simulink library "ammclib_bam_S32K3xx"  (R2016a)
settings: Solver=VariableStepAuto  SolverMode=SingleTasking  StartTime=0.0  StopTime=10.0  RelTol=1e-3
undefined symbols (not defined in the file or in its folder): a1, a2, ADCMaxError, autoCalcEn, b0, b1, b2, cfg, dgain, escale, f16A1, f16A2, f16ADCMaxError, f16B0, f16B1, f16B2, f16C1, f16CC1sc, f16CC1sc_D, f16CC1sc_Q, f16CC2sc, f16CC2sc_D, f16CC2sc_Q, f16DerivGain, f16EGain, f16FiltCoef, f16HystOff, f16HystOn, f16IGain, f16IntegGain, f16IntegGain_D, f16IntegGain_Q, f16IntegGainQ, f16Kd, f16KLs, f16Kq, f16KRs, f16Limit, f16LowerLimit, f16LowerLimit_D, f16LowerLimit_Q, f16LowerLimitQ, f16ModIndex, f16OutValOff, f16OutValOn, f16PropGain, f16PropGain_D, f16PropGain_Q, f16PropGainQ, f16RampDown, f16RampUp, f16UGain, f16UpperLimit, f16UpperLimit_D, f16UpperLimit_Q, f16UpperLimitQ, f16WIGain, f32A1, f32A2, f32ADCMaxError ... (+180)
(part 48 of 50)

== system ammclib_bam_S32K3xx/GMCLIB/F32/GMCLIB_SvmU0n_F32 ==
  pIn : Inport  OutDataTypeStr=Bus: SWLIBS_2Syst_F32  BusOutputAsStruct=on
  GMCLIB_SvmU0n_SF : S-Function  FunctionName=GMCLIB_SvmU0n_SF_F32  SFunctionDeploymentMode=off  EnableBusSupport=off
  copyright : Subsystem
      mask Display: text(10,90,'FILE:');text(10,75,'DESRIPTION:');text(10,60,'COPYRIGHT:');text(10,45,'VERSION:');text(10,30,'DATE:')
  copyright2 : Subsystem
      mask Display: text(10,90,'GMCLIB_SvmU0n_BAM_F32.slx');text(10,75,'Special Space Vector Modulation with O_000 Nulls.');text(10,60,'NXP 2022');text(10,45,'1.0');text(10,30,'20-Apr-2022');
  u32Sector : Outport
  pOut : Outport  Port=2
  wires:
  GMCLIB_SvmU0n_SF/2 -> pOut/1
  GMCLIB_SvmU0n_SF/1 -> u32Sector/1
  pIn/1 -> GMCLIB_SvmU0n_SF/1

== system ammclib_bam_S32K3xx/GMCLIB/F32/GMCLIB_SvmU7n_F32 ==
  pIn : Inport  OutDataTypeStr=Bus: SWLIBS_2Syst_F32  BusOutputAsStruct=on
  GMCLIB_SvmU7n_SF : S-Function  FunctionName=GMCLIB_SvmU7n_SF_F32  SFunctionDeploymentMode=off  EnableBusSupport=off
  copyright : Subsystem
      mask Display: text(10,90,'FILE:');text(10,75,'DESRIPTION:');text(10,60,'COPYRIGHT:');text(10,45,'VERSION:');text(10,30,'DATE:')
  copyright2 : Subsystem
      mask Display: text(10,90,'GMCLIB_SvmU7n_BAM_F32.slx');text(10,75,'Special Space Vector Modulation with O_111 Ones.');text(10,60,'NXP 2022');text(10,45,'1.0');text(10,30,'20-Apr-2022');
  u32Sector : Outport
  pOut : Outport  Port=2
  wires:
  GMCLIB_SvmU7n_SF/2 -> pOut/1
  GMCLIB_SvmU7n_SF/1 -> u32Sector/1
  pIn/1 -> GMCLIB_SvmU7n_SF/1

== system ammclib_bam_S32K3xx/GMCLIB/F32/GMCLIB_VRot_F32 ==
  f32InVec : Inport  OutDataTypeStr=Bus: SWLIBS_2Syst_F32  BusOutputAsStruct=on
  f32Angle : Inport  Port=2  OutDataTypeStr=int32
  GMCLIB_VRot_SF : S-Function  FunctionName=GMCLIB_VRot_SF_F32  SFunctionDeploymentMode=off  EnableBusSupport=off
  copyright : Subsystem
      mask Display: text(10,90,'FILE:');text(10,75,'DESRIPTION:');text(10,60,'COPYRIGHT:');text(10,45,'VERSION:');text(10,30,'DATE:')
  copyright2 : Subsystem
      mask Display: text(10,90,'GMCLIB_VRot_BAM_F32.slx');text(10,75,'Vector rotation.');text(10,60,'NXP 2022');text(10,45,'1.0');text(10,30,'20-Apr-2022');
  f32OutVec : Outport
  wires:
  GMCLIB_VRot_SF/1 -> f32OutVec/1
  f32Angle/1 -> GMCLIB_VRot_SF/2
  f32InVec/1 -> GMCLIB_VRot_SF/1

== system ammclib_bam_S32K3xx/GMCLIB/F32/GMCLIB_VUnit_F32 ==
  f32InVec : Inport  OutDataTypeStr=Bus: SWLIBS_2Syst_F32  BusOutputAsStruct=on
  GMCLIB_VUnit_SF : S-Function  FunctionName=GMCLIB_VUnit_SF_F32  SFunctionDeploymentMode=off  EnableBusSupport=off
  copyright : Subsystem
      mask Display: text(10,90,'FILE:');text(10,75,'DESRIPTION:');text(10,60,'COPYRIGHT:');text(10,45,'VERSION:');text(10,30,'DATE:')
  copyright2 : Subsystem
      mask Display: text(10,90,'GMCLIB_VUnit_BAM_F32.slx');text(10,75,'Vector normalization.');text(10,60,'NXP 2022');text(10,45,'1.0');text(10,30,'20-Apr-2022');
  f32OutVec : Outport
  wires:
  GMCLIB_VUnit_SF/1 -> f32OutVec/1
  f32InVec/1 -> GMCLIB_VUnit_SF/1

== system ammclib_bam_S32K3xx/GMCLIB/F32/GMCLIB_Vmag2coord_F32 ==
  f32InMag : Inport  OutDataTypeStr=int32
  f32InCoord : Inport  Port=2  OutDataTypeStr=int32
  GMCLIB_Vmag2coord_SF : S-Function  FunctionName=GMCLIB_Vmag2coord_SF_F32  SFunctionDeploymentMode=off  EnableBusSupport=off
  copyright : Subsystem
      mask Display: text(10,90,'FILE:');text(10,75,'DESRIPTION:');text(10,60,'COPYRIGHT:');text(10,45,'VERSION:');text(10,30,'DATE:')
  copyright2 : Subsystem
      mask Display: text(10,90,'GMCLIB_Vmag2coord_BAM_F32.slx');text(10,75,'Calculation of the coordinate out of the magnitute and second coordinate.');text(10,60,'NXP 2022');text(10,45,'1.0');text(10,30,'20-Apr-2022');
  f32OutCoord : Outport
  wires:
  GMCLIB_Vmag2coord_SF/1 -> f32OutCoord/1
  f32InCoord/1 -> GMCLIB_Vmag2coord_SF/2
  f32InMag/1 -> GMCLIB_Vmag2coord_SF/1

== system ammclib_bam_S32K3xx/GMCLIB/F32/GMCLIB_Vpol2xy_F32 ==
  f32InVec : Inport  OutDataTypeStr=Bus: SWLIBS_2Syst_F32  BusOutputAsStruct=on
  GMCLIB_Vpol2xy_SF : S-Function  FunctionName=GMCLIB_Vpol2xy_SF_F32  SFunctionDeploymentMode=off  EnableBusSupport=off
  copyright : Subsystem
      mask Display: text(10,90,'FILE:');text(10,75,'DESRIPTION:');text(10,60,'COPYRIGHT:');text(10,45,'VERSION:');text(10,30,'DATE:')
  copyright2 : Subsystem
      mask Display: text(10,90,'GMCLIB_Vpol2xy_BAM_F32.slx');text(10,75,'Transformation of polar coordinate system to Cartesian.');text(10,60,'NXP 2022');text(10,45,'1.0');text(10,30,'20-Apr-2022');
  f32OutVec : Outport
  wires:
  GMCLIB_Vpol2xy_SF/1 -> f32OutVec/1
  f32InVec/1 -> GMCLIB_Vpol2xy_SF/1

== system ammclib_bam_S32K3xx/GMCLIB/F32/GMCLIB_Vxy2pol_F32 ==
  f32InVec : Inport  OutDataTypeStr=Bus: SWLIBS_2Syst_F32  BusOutputAsStruct=on
  GMCLIB_Vxy2pol_SF : S-Function  FunctionName=GMCLIB_Vxy2pol_SF_F32  SFunctionDeploymentMode=off  EnableBusSupport=off
  copyright : Subsystem
      mask Display: text(10,90,'FILE:');text(10,75,'DESRIPTION:');text(10,60,'COPYRIGHT:');text(10,45,'VERSION:');text(10,30,'DATE:')
  copyright2 : Subsystem
      mask Display: text(10,90,'GMCLIB_Vxy2pol_BAM_F32.slx');text(10,75,'Transformation of Cartesian coordinate system to polar.');text(10,60,'NXP 2022');text(10,45,'1.0');text(10,30,'20-Apr-2022');
  f32OutVec : Outport
  wires:
  GMCLIB_Vxy2pol_SF/1 -> f32OutVec/1
  f32InVec/1 -> GMCLIB_Vxy2pol_SF/1

== system ammclib_bam_S32K3xx/GMCLIB/FLT/GMCLIB_BetaProjection3Ph_FLT ==
  pIn : Inport  OutDataTypeStr=Bus: SWLIBS_3Syst_FLT  BusOutputAsStruct=on
  GMCLIB_BetaProjection3Ph_SF : S-Function  FunctionName=GMCLIB_BetaProjection3Ph_SF_FLT  SFunctionDeploymentMode=off  EnableBusSupport=off
  copyright : Subsystem
      mask Display: text(10,90,'FILE:');text(10,75,'DESRIPTION:');text(10,60,'COPYRIGHT:');text(10,45,'VERSION:');text(10,30,'DATE:')
  copyright2 : Subsystem
      mask Display: text(10,90,'GMCLIB_BetaProjection3Ph_BAM_FLT.slx');text(10,75,'Beta Projection transformation.');text(10,60,'NXP 2022');text(10,45,'1.0');text(10,30,'20-Apr-2022');
  pOut : Outport
  wires:
  GMCLIB_BetaProjection3Ph_SF/1 -> pOut/1
  pIn/1 -> GMCLIB_BetaProjection3Ph_SF/1

== system ammclib_bam_S32K3xx/GMCLIB/FLT/GMCLIB_BetaProjection_FLT ==
  pIn : Inport  OutDataTypeStr=Bus: SWLIBS_3Syst_FLT  BusOutputAsStruct=on
  GMCLIB_BetaProjection_SF : S-Function  FunctionName=GMCLIB_BetaProjection_SF_FLT  SFunctionDeploymentMode=off  EnableBusSupport=off
  copyright : Subsystem
      mask Display: text(10,90,'FILE:');text(10,75,'DESRIPTION:');text(10,60,'COPYRIGHT:');text(10,45,'VERSION:');text(10,30,'DATE:')
  copyright2 : Subsystem
      mask Display: text(10,90,'GMCLIB_BetaProjection_BAM_FLT.slx');text(10,75,'Beta Projection transformation.');text(10,60,'NXP 2022');text(10,45,'1.0');text(10,30,'20-Apr-2022');
  pOut : Outport
  wires:
  GMCLIB_BetaProjection_SF/1 -> pOut/1
  pIn/1 -> GMCLIB_BetaProjection_SF/1

== system ammclib_bam_S32K3xx/GMCLIB/FLT/GMCLIB_Clark6Ph_FLT ==
  pIn : Inport  OutDataTypeStr=Bus: SWLIBS_6Syst_FLT  BusOutputAsStruct=on
  GMCLIB_Clark6Ph_SF : S-Function  FunctionName=GMCLIB_Clark6Ph_SF_FLT  Parameters=fltWindingShift  SFunctionDeploymentMode=off  EnableBusSupport=off
  copyright : Subsystem
      mask Display: text(10,90,'FILE:');text(10,75,'DESRIPTION:');text(10,60,'COPYRIGHT:');text(10,45,'VERSION:');text(10,30,'DATE:')
  copyright2 : Subsystem
      mask Display: text(10,90,'GMCLIB_Clark6Ph_BAM_FLT.slx');text(10,75,'Direct 6-phase Clark transformation.');text(10,60,'NXP 2022');text(10,45,'1.0');text(10,30,'20-Apr-2022');
  pOut : Outport
  wires:
  GMCLIB_Clark6Ph_SF/1 -> pOut/1
  pIn/1 -> GMCLIB_Clark6Ph_SF/1

== system ammclib_bam_S32K3xx/GMCLIB/FLT/GMCLIB_ClarkInv6Ph_FLT ==
  pIn : Inport  OutDataTypeStr=Bus: SWLIBS_2Syst_FLT  BusOutputAsStruct=on
  GMCLIB_ClarkInv6Ph_SF : S-Function  FunctionName=GMCLIB_ClarkInv6Ph_SF_FLT  Parameters=fltWindingShift  SFunctionDeploymentMode=off  EnableBusSupport=off
  copyright : Subsystem
      mask Display: text(10,90,'FILE:');text(10,75,'DESRIPTION:');text(10,60,'COPYRIGHT:');text(10,45,'VERSION:');text(10,30,'DATE:')
  copyright2 : Subsystem
      mask Display: text(10,90,'GMCLIB_ClarkInv6Ph_BAM_FLT.slx');text(10,75,'Inverse Clarke transform for six-phase systems.');text(10,60,'NXP 2022');text(10,45,'1.0');text(10,30,'20-Apr-2022');
  pOut : Outport
  wires:
  GMCLIB_ClarkInv6Ph_SF/1 -> pOut/1
  pIn/1 -> GMCLIB_ClarkInv6Ph_SF/1

== system ammclib_bam_S32K3xx/GMCLIB/FLT/GMCLIB_ClarkInv_FLT ==
  pIn : Inport  OutDataTypeStr=Bus: SWLIBS_2Syst_FLT  BusOutputAsStruct=on
  GMCLIB_ClarkInv_SF : S-Function  FunctionName=GMCLIB_ClarkInv_SF_FLT  SFunctionDeploymentMode=off  EnableBusSupport=off
  copyright : Subsystem
      mask Display: text(10,90,'FILE:');text(10,75,'DESRIPTION:');text(10,60,'COPYRIGHT:');text(10,45,'VERSION:');text(10,30,'DATE:')
  copyright2 : Subsystem
      mask Display: text(10,90,'GMCLIB_ClarkInv_BAM_FLT.slx');text(10,75,'Inverse Clarke transformation');text(10,60,'NXP 2022');text(10,45,'1.0');text(10,30,'20-Apr-2022');
  pOut : Outport
  wires:
  GMCLIB_ClarkInv_SF/1 -> pOut/1
  pIn/1 -> GMCLIB_ClarkInv_SF/1

== system ammclib_bam_S32K3xx/GMCLIB/FLT/GMCLIB_Clark_FLT ==
  pIn : Inport  OutDataTypeStr=Bus: SWLIBS_3Syst_FLT  BusOutputAsStruct=on
  GMCLIB_Clark_SF : S-Function  FunctionName=GMCLIB_Clark_SF_FLT  SFunctionDeploymentMode=off  EnableBusSupport=off
  copyright : Subsystem
      mask Display: text(10,90,'FILE:');text(10,75,'DESRIPTION:');text(10,60,'COPYRIGHT:');text(10,45,'VERSION:');text(10,30,'DATE:')
  copyright2 : Subsystem
      mask Display: text(10,90,'GMCLIB_Clark_BAM_FLT.slx');text(10,75,'Clarke transformation.');text(10,60,'NXP 2022');text(10,45,'1.0');text(10,30,'20-Apr-2022');
  pOut : Outport
  wires:
  GMCLIB_Clark_SF/1 -> pOut/1
  pIn/1 -> GMCLIB_Clark_SF/1

== system ammclib_bam_S32K3xx/GMCLIB/FLT/GMCLIB_DecouplingPMSM_FLT ==
  pUdq : Inport  OutDataTypeStr=Bus: SWLIBS_2Syst_FLT  BusOutputAsStruct=on
  pIdq : Inport  Port=2  OutDataTypeStr=Bus: SWLIBS_2Syst_FLT  BusOutputAsStruct=on
  fltAngularVel : Inport  Port=3  OutDataTypeStr=single
  GMCLIB_DecouplingPMSM_SF : S-Function  FunctionName=GMCLIB_DecouplingPMSM_SF_FLT  Parameters=showStates,fltLD,fltLQ  SFunctionDeploymentMode=off  EnableBusSupport=off
  copyright : Subsystem
      mask Display: text(10,90,'FILE:');text(10,75,'DESRIPTION:');text(10,60,'COPYRIGHT:');text(10,45,'VERSION:');text(10,30,'DATE:')
  copyright2 : Subsystem
      mask Display: text(10,90,'GMCLIB_DecouplingPMSM_BAM_FLT.slx');text(10,75,'Decoupling of d and q axis of PMSM model.');text(10,60,'NXP 2022');text(10,45,'1.0');text(10,30,'20-Apr-2022');
  fltLD : Ground
  fltLQ : Ground
  pUdqDec : Outport
  wires:
  GMCLIB_DecouplingPMSM_SF/1 -> pUdqDec/1
  fltLQ/1 -> GMCLIB_DecouplingPMSM_SF/5
  fltLD/1 -> GMCLIB_DecouplingPMSM_SF/4
  fltAngularVel/1 -> GMCLIB_DecouplingPMSM_SF/3
  pIdq/1 -> GMCLIB_DecouplingPMSM_SF/2
  pUdq/1 -> GMCLIB_DecouplingPMSM_SF/1

== system ammclib_bam_S32K3xx/GMCLIB/FLT/GMCLIB_ElimDcBusRip_FLT ==
  pIn : Inport  OutDataTypeStr=Bus: SWLIBS_2Syst_FLT  BusOutputAsStruct=on
  fltArgDcBusMsr : Inport  Port=2  OutDataTypeStr=single
  GMCLIB_ElimDcBusRip_SF : S-Function  FunctionName=GMCLIB_ElimDcBusRip_SF_FLT  Parameters=showStates,fltModIndex  SFunctionDeploymentMode=off  EnableBusSupport=off
  copyright : Subsystem
      mask Display: text(10,90,'FILE:');text(10,75,'DESRIPTION:');text(10,60,'COPYRIGHT:');text(10,45,'VERSION:');text(10,30,'DATE:')
  copyright2 : Subsystem
      mask Display: text(10,90,'GMCLIB_ElimDcBusRip_BAM_FLT.slx');text(10,75,'DC Bus voltage ripple elimination function.');text(10,60,'NXP 2022');text(10,45,'1.0');text(10,30,'20-Apr-2022');
  fltModIndex : Ground
  pOut : Outport
  wires:
  GMCLIB_ElimDcBusRip_SF/1 -> pOut/1
  fltModIndex/1 -> GMCLIB_ElimDcBusRip_SF/3
  fltArgDcBusMsr/1 -> GMCLIB_ElimDcBusRip_SF/2
  pIn/1 -> GMCLIB_ElimDcBusRip_SF/1

== system ammclib_bam_S32K3xx/GMCLIB/FLT/GMCLIB_ParkInv_FLT ==
  pInAngle : Inport  OutDataTypeStr=Bus: SWLIBS_2Syst_FLT  BusOutputAsStruct=on
  pIn : Inport  Port=2  OutDataTypeStr=Bus: SWLIBS_2Syst_FLT  BusOutputAsStruct=on
  GMCLIB_ParkInv_SF : S-Function  FunctionName=GMCLIB_ParkInv_SF_FLT  SFunctionDeploymentMode=off  EnableBusSupport=off
  copyright : Subsystem
      mask Display: text(10,90,'FILE:');text(10,75,'DESRIPTION:');text(10,60,'COPYRIGHT:');text(10,45,'VERSION:');text(10,30,'DATE:')
  copyright2 : Subsystem
      mask Display: text(10,90,'GMCLIB_ParkInv_BAM_FLT.slx');text(10,75,'Inverse Park transformation.');text(10,60,'NXP 2022');text(10,45,'1.0');text(10,30,'20-Apr-2022');
  pOut : Outport
  wires:
  GMCLIB_ParkInv_SF/1 -> pOut/1
  pIn/1 -> GMCLIB_ParkInv_SF/2
  pInAngle/1 -> GMCLIB_ParkInv_SF/1

== system ammclib_bam_S32K3xx/GMCLIB/FLT/GMCLIB_Park_FLT ==
  pInAngle : Inport  OutDataTypeStr=Bus: SWLIBS_2Syst_FLT  BusOutputAsStruct=on
  pIn : Inport  Port=2  OutDataTypeStr=Bus: SWLIBS_2Syst_FLT  BusOutputAsStruct=on
  GMCLIB_Park_SF : S-Function  FunctionName=GMCLIB_Park_SF_FLT  SFunctionDeploymentMode=off  EnableBusSupport=off
  copyright : Subsystem
      mask Display: text(10,90,'FILE:');text(10,75,'DESRIPTION:');text(10,60,'COPYRIGHT:');text(10,45,'VERSION:');text(10,30,'DATE:')
  copyright2 : Subsystem
      mask Display: text(10,90,'GMCLIB_Park_BAM_FLT.slx');text(10,75,'Park transformation.');text(10,60,'NXP 2022');text(10,45,'1.0');text(10,30,'20-Apr-2022');
  pOut : Outport
  wires:
  GMCLIB_Park_SF/1 -> pOut/1
  pIn/1 -> GMCLIB_Park_SF/2
  pInAngle/1 -> GMCLIB_Park_SF/1

== system ammclib_bam_S32K3xx/GMCLIB/FLT/GMCLIB_PwmIct_FLT ==
  pIn : Inport  OutDataTypeStr=Bus: SWLIBS_2Syst_FLT  BusOutputAsStruct=on
  GMCLIB_PwmIct_SF : S-Function  FunctionName=GMCLIB_PwmIct_SF_FLT  SFunctionDeploymentMode=off  EnableBusSupport=off
  copyright : Subsystem
      mask Display: text(10,90,'FILE:');text(10,75,'DESRIPTION:');text(10,60,'COPYRIGHT:');text(10,45,'VERSION:');text(10,30,'DATE:')
  copyright2 : Subsystem
      mask Display: text(10,90,'GMCLIB_PwmIct_BAM_FLT.slx');text(10,75,'General Sinusoidal PWM.');text(10,60,'NXP 2022');text(10,45,'1.0');text(10,30,'20-Apr-2022');
  u32Sector : Outport
  pOut : Outport  Port=2
  wires:
  GMCLIB_PwmIct_SF/2 -> pOut/1
  GMCLIB_PwmIct_SF/1 -> u32Sector/1
  pIn/1 -> GMCLIB_PwmIct_SF/1

== system ammclib_bam_S32K3xx/GMCLIB/FLT/GMCLIB_SvmSci_FLT ==
  pIn : Inport  OutDataTypeStr=Bus: SWLIBS_2Syst_FLT  BusOutputAsStruct=on
  GMCLIB_SvmSci_SF : S-Function  FunctionName=GMCLIB_SvmSci_SF_FLT  SFunctionDeploymentMode=off  EnableBusSupport=off
  copyright : Subsystem
      mask Display: text(10,90,'FILE:');text(10,75,'DESRIPTION:');text(10,60,'COPYRIGHT:');text(10,45,'VERSION:');text(10,30,'DATE:')
  copyright2 : Subsystem
      mask Display: text(10,90,'GMCLIB_SvmSci_BAM_FLT.slx');text(10,75,'General Sinusoidal Modulation with Injection of Third Harmonic.');text(10,60,'NXP 2022');text(10,45,'1.0');text(10,30,'20-Apr-2022');
  u32Sector : Outport
  pOut : Outport  Port=2
  wires:
  GMCLIB_SvmSci_SF/2 -> pOut/1
  GMCLIB_SvmSci_SF/1 -> u32Sector/1
  pIn/1 -> GMCLIB_SvmSci_SF/1

== system ammclib_bam_S32K3xx/GMCLIB/FLT/GMCLIB_SvmStd6Ph_FLT ==
  pIn : Inport  OutDataTypeStr=Bus: SWLIBS_2Syst_FLT  BusOutputAsStruct=on
  GMCLIB_SvmStd6Ph_SF : S-Function  FunctionName=GMCLIB_SvmStd6Ph_SF_FLT  Parameters=fltWindingShift  SFunctionDeploymentMode=off  EnableBusSupport=off
  copyright : Subsystem
      mask Display: text(10,90,'FILE:');text(10,75,'DESRIPTION:');text(10,60,'COPYRIGHT:');text(10,45,'VERSION:');text(10,30,'DATE:')
  copyright2 : Subsystem
      mask Display: text(10,90,'GMCLIB_SvmStd6Ph_BAM_FLT.slx');text(10,75,'Six-phase Space Vector Modulation.');text(10,60,'NXP 2022');text(10,45,'1.0');text(10,30,'20-Apr-2022');
  pOut : Outport
  pOutSector : Outport  Port=2
  wires:
  GMCLIB_SvmStd6Ph_SF/2 -> pOutSector/1
  GMCLIB_SvmStd6Ph_SF/1 -> pOut/1
  pIn/1 -> GMCLIB_SvmStd6Ph_SF/1

== system ammclib_bam_S32K3xx/GMCLIB/FLT/GMCLIB_SvmStd_FLT ==
  pIn : Inport  OutDataTypeStr=Bus: SWLIBS_2Syst_FLT  BusOutputAsStruct=on
  GMCLIB_SvmStd_SF : S-Function  FunctionName=GMCLIB_SvmStd_SF_FLT  SFunctionDeploymentMode=off  EnableBusSupport=off
  copyright : Subsystem
      mask Display: text(10,90,'FILE:');text(10,75,'DESRIPTION:');text(10,60,'COPYRIGHT:');text(10,45,'VERSION:');text(10,30,'DATE:')
  copyright2 : Subsystem
      mask Display: text(10,90,'GMCLIB_SvmStd_BAM_FLT.slx');text(10,75,'Standard Space Vector Modulation.');text(10,60,'NXP 2022');text(10,45,'1.0');text(10,30,'20-Apr-2022');
  u32Sector : Outport
  pOut : Outport  Port=2
  wires:
  GMCLIB_SvmStd_SF/2 -> pOut/1
  GMCLIB_SvmStd_SF/1 -> u32Sector/1
  pIn/1 -> GMCLIB_SvmStd_SF/1

== system ammclib_bam_S32K3xx/GMCLIB/FLT/GMCLIB_SvmU0n_FLT ==
  pIn : Inport  OutDataTypeStr=Bus: SWLIBS_2Syst_FLT  BusOutputAsStruct=on
  GMCLIB_SvmU0n_SF : S-Function  FunctionName=GMCLIB_SvmU0n_SF_FLT  SFunctionDeploymentMode=off  EnableBusSupport=off
  copyright : Subsystem
      mask Display: text(10,90,'FILE:');text(10,75,'DESRIPTION:');text(10,60,'COPYRIGHT:');text(10,45,'VERSION:');text(10,30,'DATE:')
  copyright2 : Subsystem
      mask Display: text(10,90,'GMCLIB_SvmU0n_BAM_FLT.slx');text(10,75,'Special Space Vector Modulation with O_000 Nulls.');text(10,60,'NXP 2022');text(10,45,'1.0');text(10,30,'20-Apr-2022');
  u32Sector : Outport
  pOut : Outport  Port=2
  wires:
  GMCLIB_SvmU0n_SF/2 -> pOut/1
  GMCLIB_SvmU0n_SF/1 -> u32Sector/1
  pIn/1 -> GMCLIB_SvmU0n_SF/1

== system ammclib_bam_S32K3xx/GMCLIB/FLT/GMCLIB_SvmU7n_FLT ==
  pIn : Inport  OutDataTypeStr=Bus: SWLIBS_2Syst_FLT  BusOutputAsStruct=on
  GMCLIB_SvmU7n_SF : S-Function  FunctionName=GMCLIB_SvmU7n_SF_FLT  SFunctionDeploymentMode=off  EnableBusSupport=off
  copyright : Subsystem
      mask Display: text(10,90,'FILE:');text(10,75,'DESRIPTION:');text(10,60,'COPYRIGHT:');text(10,45,'VERSION:');text(10,30,'DATE:')
  copyright2 : Subsystem
      mask Display: text(10,90,'GMCLIB_SvmU7n_BAM_FLT.slx');text(10,75,'Special Space Vector Modulation with O_111 Ones.');text(10,60,'NXP 2022');text(10,45,'1.0');text(10,30,'20-Apr-2022');
  u32Sector : Outport
  pOut : Outport  Port=2
  wires:
  GMCLIB_SvmU7n_SF/2 -> pOut/1
  GMCLIB_SvmU7n_SF/1 -> u32Sector/1
  pIn/1 -> GMCLIB_SvmU7n_SF/1

== system ammclib_bam_S32K3xx/GMCLIB/FLT/GMCLIB_VRot_FLT ==
  fltInVec : Inport  OutDataTypeStr=Bus: SWLIBS_2Syst_FLT  BusOutputAsStruct=on
  fltAngle : Inport  Port=2  OutDataTypeStr=single
  GMCLIB_VRot_SF : S-Function  FunctionName=GMCLIB_VRot_SF_FLT  SFunctionDeploymentMode=off  EnableBusSupport=off
  copyright : Subsystem
      mask Display: text(10,90,'FILE:');text(10,75,'DESRIPTION:');text(10,60,'COPYRIGHT:');text(10,45,'VERSION:');text(10,30,'DATE:')
  copyright2 : Subsystem
      mask Display: text(10,90,'GMCLIB_VRot_BAM_FLT.slx');text(10,75,'Vector rotation.');text(10,60,'NXP 2022');text(10,45,'1.0');text(10,30,'20-Apr-2022');
  fltOutVec : Outport
  wires:
  GMCLIB_VRot_SF/1 -> fltOutVec/1
  fltAngle/1 -> GMCLIB_VRot_SF/2
  fltInVec/1 -> GMCLIB_VRot_SF/1

== system ammclib_bam_S32K3xx/GMCLIB/FLT/GMCLIB_VUnit_FLT ==
  fltInVec : Inport  OutDataTypeStr=Bus: SWLIBS_2Syst_FLT  BusOutputAsStruct=on
  GMCLIB_VUnit_SF : S-Function  FunctionName=GMCLIB_VUnit_SF_FLT  SFunctionDeploymentMode=off  EnableBusSupport=off
  copyright : Subsystem
      mask Display: text(10,90,'FILE:');text(10,75,'DESRIPTION:');text(10,60,'COPYRIGHT:');text(10,45,'VERSION:');text(10,30,'DATE:')
  copyright2 : Subsystem
      mask Display: text(10,90,'GMCLIB_VUnit_BAM_FLT.slx');text(10,75,'Vector normalization.');text(10,60,'NXP 2022');text(10,45,'1.0');text(10,30,'20-Apr-2022');
  fltOutVec : Outport
  wires:
  GMCLIB_VUnit_SF/1 -> fltOutVec/1
  fltInVec/1 -> GMCLIB_VUnit_SF/1

== system ammclib_bam_S32K3xx/GMCLIB/FLT/GMCLIB_Vmag2coord_FLT ==
  fltInMag : Inport  OutDataTypeStr=single
  fltInCoord : Inport  Port=2  OutDataTypeStr=single
  GMCLIB_Vmag2coord_SF : S-Function  FunctionName=GMCLIB_Vmag2coord_SF_FLT  SFunctionDeploymentMode=off  EnableBusSupport=off
  copyright : Subsystem
      mask Display: text(10,90,'FILE:');text(10,75,'DESRIPTION:');text(10,60,'COPYRIGHT:');text(10,45,'VERSION:');text(10,30,'DATE:')
  copyright2 : Subsystem
      mask Display: text(10,90,'GMCLIB_Vmag2coord_BAM_FLT.slx');text(10,75,'Calculation of the coordinate out of the magnitute and second coordinate.');text(10,60,'NXP 2022');text(10,45,'1.0');text(10,30,'20-Apr-2022');
  fltOutCoord : Outport
  wires:
  GMCLIB_Vmag2coord_SF/1 -> fltOutCoord/1
  fltInCoord/1 -> GMCLIB_Vmag2coord_SF/2
  fltInMag/1 -> GMCLIB_Vmag2coord_SF/1

== system ammclib_bam_S32K3xx/GMCLIB/FLT/GMCLIB_Vpol2xy_FLT ==
  fltInVec : Inport  OutDataTypeStr=Bus: SWLIBS_2Syst_FLT  BusOutputAsStruct=on
  GMCLIB_Vpol2xy_SF : S-Function  FunctionName=GMCLIB_Vpol2xy_SF_FLT  SFunctionDeploymentMode=off  EnableBusSupport=off
  copyright : Subsystem
      mask Display: text(10,90,'FILE:');text(10,75,'DESRIPTION:');text(10,60,'COPYRIGHT:');text(10,45,'VERSION:');text(10,30,'DATE:')
  copyright2 : Subsystem
      mask Display: text(10,90,'GMCLIB_Vpol2xy_BAM_FLT.slx');text(10,75,'Transformation of polar coordinate system to Cartesian.');text(10,60,'NXP 2022');text(10,45,'1.0');text(10,30,'20-Apr-2022');
  fltOutVec : Outport
  wires:
  GMCLIB_Vpol2xy_SF/1 -> fltOutVec/1
  fltInVec/1 -> GMCLIB_Vpol2xy_SF/1

== system ammclib_bam_S32K3xx/GMCLIB/FLT/GMCLIB_Vxy2pol_FLT ==
  fltInVec : Inport  OutDataTypeStr=Bus: SWLIBS_2Syst_FLT  BusOutputAsStruct=on
  GMCLIB_Vxy2pol_SF : S-Function  FunctionName=GMCLIB_Vxy2pol_SF_FLT  SFunctionDeploymentMode=off  EnableBusSupport=off
  copyright : Subsystem
      mask Display: text(10,90,'FILE:');text(10,75,'DESRIPTION:');text(10,60,'COPYRIGHT:');text(10,45,'VERSION:');text(10,30,'DATE:')
  copyright2 : Subsystem
      mask Display: text(10,90,'GMCLIB_Vxy2pol_BAM_FLT.slx');text(10,75,'Transformation of Cartesian coordinate system to polar.');text(10,60,'NXP 2022');text(10,45,'1.0');text(10,30,'20-Apr-2022');
  fltOutVec : Outport
  wires:
  GMCLIB_Vxy2pol_SF/1 -> fltOutVec/1
  fltInVec/1 -> GMCLIB_Vxy2pol_SF/1

== system ammclib_bam_S32K3xx/GMCLIB/Generic/GMCLIB_SpreadPWM ==
  GMCLIB_SpreadPWM_SF : S-Function  FunctionName=GMCLIB_SpreadPWM_SF  Parameters=u32PWMFreq,u16Mod,u32SpreadFreq,u8FreqDev  SFunctionDeploymentMode=off  EnableBusSupport=off
  copyright : Subsystem
      mask Display: text(10,90,'FILE:');text(10,75,'DESRIPTION:');text(10,60,'COPYRIGHT:');text(10,45,'VERSION:');text(10,30,'DATE:')
  copyright2 : Subsystem
      mask Display: text(10,90,'GMCLIB_SpreadPWM_BAM.slx');text(10,75,'Spreading sequence generator');text(10,60,'NXP 2022');text(10,45,'1.0');text(10,30,'20-Apr-2022');
  u16Modulus : Outport
  wires:
  GMCLIB_SpreadPWM_SF/1 -> u16Modulus/1

== system ammclib_bam_S32K3xx/MLIB/F16/MLIB_AbsSat_F16 ==
  f16In : Inport  OutDataTypeStr=int16
  MLIB_AbsSat_SF : S-Function  FunctionName=MLIB_AbsSat_SF_F16  SFunctionDeploymentMode=off  EnableBusSupport=off
  copyright : Subsystem
      mask Display: text(10,90,'FILE:');text(10,75,'DESRIPTION:');text(10,60,'COPYRIGHT:');text(10,45,'VERSION:');text(10,30,'DATE:')
  copyright2 : Subsystem
      mask Display: text(10,90,'MLIB_AbsSat_BAM_F16.slx');text(10,75,'Saturated absolute value.');text(10,60,'NXP 2022');text(10,45,'1.0');text(10,30,'20-Apr-2022');
  f16Out : Outport
  wires:
  MLIB_AbsSat_SF/1 -> f16Out/1
  f16In/1 -> MLIB_AbsSat_SF/1

== system ammclib_bam_S32K3xx/MLIB/F16/MLIB_Abs_F16 ==
  f16In : Inport  OutDataTypeStr=int16
  MLIB_Abs_SF : S-Function  FunctionName=MLIB_Abs_SF_F16  SFunctionDeploymentMode=off  EnableBusSupport=off
  copyright : Subsystem
      mask Display: text(10,90,'FILE:');text(10,75,'DESRIPTION:');text(10,60,'COPYRIGHT:');text(10,45,'VERSION:');text(10,30,'DATE:')
  copyright2 : Subsystem
      mask Display: text(10,90,'MLIB_Abs_BAM_F16.slx');text(10,75,'Unsaturated absolute value.');text(10,60,'NXP 2022');text(10,45,'1.0');text(10,30,'20-Apr-2022');
  f16Out : Outport
  wires:
  MLIB_Abs_SF/1 -> f16Out/1
  f16In/1 -> MLIB_Abs_SF/1

== system ammclib_bam_S32K3xx/MLIB/F16/MLIB_AddSat_F16 ==
  f16In1 : Inport  OutDataTypeStr=int16
  f16In2 : Inport  Port=2  OutDataTypeStr=int16
  MLIB_AddSat_SF : S-Function  FunctionName=MLIB_AddSat_SF_F16  SFunctionDeploymentMode=off  EnableBusSupport=off
  copyright : Subsystem
      mask Display: text(10,90,'FILE:');text(10,75,'DESRIPTION:');text(10,60,'COPYRIGHT:');text(10,45,'VERSION:');text(10,30,'DATE:')
  copyright2 : Subsystem
      mask Display: text(10,90,'MLIB_AddSat_BAM_F16.slx');text(10,75,'Saturated addition.');text(10,60,'NXP 2022');text(10,45,'1.0');text(10,30,'20-Apr-2022');
  f16Out : Outport
  wires:
  MLIB_AddSat_SF/1 -> f16Out/1
  f16In2/1 -> MLIB_AddSat_SF/2
  f16In1/1 -> MLIB_AddSat_SF/1

== system ammclib_bam_S32K3xx/MLIB/F16/MLIB_Add_F16 ==
  f16In1 : Inport  OutDataTypeStr=int16
  f16In2 : Inport  Port=2  OutDataTypeStr=int16
  MLIB_Add_SF : S-Function  FunctionName=MLIB_Add_SF_F16  SFunctionDeploymentMode=off  EnableBusSupport=off
  copyright : Subsystem
      mask Display: text(10,90,'FILE:');text(10,75,'DESRIPTION:');text(10,60,'COPYRIGHT:');text(10,45,'VERSION:');text(10,30,'DATE:')
  copyright2 : Subsystem
      mask Display: text(10,90,'MLIB_Add_BAM_F16.slx');text(10,75,'Unsaturated addition.');text(10,60,'NXP 2022');text(10,45,'1.0');text(10,30,'20-Apr-2022');
  f16Out : Outport
  wires:
  MLIB_Add_SF/1 -> f16Out/1
  f16In2/1 -> MLIB_Add_SF/2
  f16In1/1 -> MLIB_Add_SF/1

== system ammclib_bam_S32K3xx/MLIB/F16/MLIB_ConvertPU_F16F32 ==
  f32In : Inport  OutDataTypeStr=int32
  MLIB_ConvertPU_SF : S-Function  FunctionName=MLIB_ConvertPU_SF_F16F32  SFunctionDeploymentMode=off  EnableBusSupport=off
  copyright : Subsystem
      mask Display: text(10,90,'FILE:');text(10,75,'DESRIPTION:');text(10,60,'COPYRIGHT:');text(10,45,'VERSION:');text(10,30,'DATE:')
  copyright2 : Subsystem
      mask Display: text(10,90,'MLIB_ConvertPU_BAM_F16F32.slx');text(10,75,'Converts the input value to a different representation.');text(10,60,'NXP 2022');text(10,45,'1.0');text(10,30,'20-Apr-2022');
  f16Out : Outport
  wires:
  MLIB_ConvertPU_SF/1 -> f16Out/1
  f32In/1 -> MLIB_ConvertPU_SF/1

== system ammclib_bam_S32K3xx/MLIB/F16/MLIB_ConvertPU_F16FLT ==
  fltIn : Inport  OutDataTypeStr=single
  MLIB_ConvertPU_SF : S-Function  FunctionName=MLIB_ConvertPU_SF_F16FLT  SFunctionDeploymentMode=off  EnableBusSupport=off
  copyright : Subsystem
      mask Display: text(10,90,'FILE:');text(10,75,'DESRIPTION:');text(10,60,'COPYRIGHT:');text(10,45,'VERSION:');text(10,30,'DATE:')
  copyright2 : Subsystem
      mask Display: text(10,90,'MLIB_ConvertPU_BAM_F16FLT.slx');text(10,75,'Converts the input value to a different representation.');text(10,60,'NXP 2022');text(10,45,'1.0');text(10,30,'20-Apr-2022');
  f16Out : Outport
  wires:
  MLIB_ConvertPU_SF/1 -> f16Out/1
  fltIn/1 -> MLIB_ConvertPU_SF/1

== system ammclib_bam_S32K3xx/MLIB/F16/MLIB_Convert_F16F32 ==
  f32In1 : Inport  OutDataTypeStr=int32
  f32In2 : Inport  Port=2  OutDataTypeStr=int32
  MLIB_Convert_SF : S-Function  FunctionName=MLIB_Convert_SF_F16F32  SFunctionDeploymentMode=off  EnableBusSupport=off
  copyright : Subsystem
      mask Display: text(10,90,'FILE:');text(10,75,'DESRIPTION:');text(10,60,'COPYRIGHT:');text(10,45,'VERSION:');text(10,30,'DATE:')
  copyright2 : Subsystem
      mask Display: text(10,90,'MLIB_Convert_BAM_F16F32.slx');text(10,75,'Converts the input value with scale to a different representation.');text(10,60,'NXP 2022');text(10,45,'1.0');text(10,30,'20-Apr-2022');
  f16Out : Outport
  wires:
  MLIB_Convert_SF/1 -> f16Out/1
  f32In2/1 -> MLIB_Convert_SF/2
  f32In1/1 -> MLIB_Convert_SF/1

== system ammclib_bam_S32K3xx/MLIB/F16/MLIB_Convert_F16FLT ==
  fltIn1 : Inport  OutDataTypeStr=single
  fltIn2 : Inport  Port=2  OutDataTypeStr=single
  MLIB_Convert_SF : S-Function  FunctionName=MLIB_Convert_SF_F16FLT  SFunctionDeploymentMode=off  EnableBusSupport=off
  copyright : Subsystem
      mask Display: text(10,90,'FILE:');text(10,75,'DESRIPTION:');text(10,60,'COPYRIGHT:');text(10,45,'VERSION:');text(10,30,'DATE:')
  copyright2 : Subsystem
      mask Display: text(10,90,'MLIB_Convert_BAM_F16FLT.slx');text(10,75,'Converts the input value with scale to a different representation.');text(10,60,'NXP 2022');text(10,45,'1.0');text(10,30,'20-Apr-2022');
  f16Out : Outport
  wires:
  MLIB_Convert_SF/1 -> f16Out/1
  fltIn2/1 -> MLIB_Convert_SF/2
  fltIn1/1 -> MLIB_Convert_SF/1

== system ammclib_bam_S32K3xx/MLIB/F16/MLIB_DivSat_F16 ==
  f16In1 : Inport  OutDataTypeStr=int16
  f16In2 : Inport  Port=2  OutDataTypeStr=int16
  MLIB_DivSat_SF : S-Function  FunctionName=MLIB_DivSat_SF_F16  SFunctionDeploymentMode=off  EnableBusSupport=off
  copyright : Subsystem
      mask Display: text(10,90,'FILE:');text(10,75,'DESRIPTION:');text(10,60,'COPYRIGHT:');text(10,45,'VERSION:');text(10,30,'DATE:')
  copyright2 : Subsystem
      mask Display: text(10,90,'MLIB_DivSat_BAM_F16.slx');text(10,75,'Saturated division.');text(10,60,'NXP 2022');text(10,45,'1.0');text(10,30,'20-Apr-2022');
  f16Out : Outport
  wires:
  MLIB_DivSat_SF/1 -> f16Out/1
  f16In2/1 -> MLIB_DivSat_SF/2
  f16In1/1 -> MLIB_DivSat_SF/1

== system ammclib_bam_S32K3xx/MLIB/F16/MLIB_Div_F16 ==
  f16In1 : Inport  OutDataTypeStr=int16
  f16In2 : Inport  Port=2  OutDataTypeStr=int16
  MLIB_Div_SF : S-Function  FunctionName=MLIB_Div_SF_F16  SFunctionDeploymentMode=off  EnableBusSupport=off
  copyright : Subsystem
      mask Display: text(10,90,'FILE:');text(10,75,'DESRIPTION:');text(10,60,'COPYRIGHT:');text(10,45,'VERSION:');text(10,30,'DATE:')
  copyright2 : Subsystem
      mask Display: text(10,90,'MLIB_Div_BAM_F16.slx');text(10,75,'Division of two input values.');text(10,60,'NXP 2022');text(10,45,'1.0');text(10,30,'20-Apr-2022');
  f16Out : Outport
  wires:
  MLIB_Div_SF/1 -> f16Out/1
  f16In2/1 -> MLIB_Div_SF/2
  f16In1/1 -> MLIB_Div_SF/1

== system ammclib_bam_S32K3xx/MLIB/F16/MLIB_MacSat_F16 ==
  f16In1 : Inport  OutDataTypeStr=int16
  f16In2 : Inport  Port=2  OutDataTypeStr=int16
  f16In3 : Inport  Port=3  OutDataTypeStr=int16
  MLIB_MacSat_SF : S-Function  FunctionName=MLIB_MacSat_SF_F16  SFunctionDeploymentMode=off  EnableBusSupport=off
  copyright : Subsystem
      mask Display: text(10,90,'FILE:');text(10,75,'DESRIPTION:');text(10,60,'COPYRIGHT:');text(10,45,'VERSION:');text(10,30,'DATE:')
  copyright2 : Subsystem
      mask Display: text(10,90,'MLIB_MacSat_BAM_F16.slx');text(10,75,'Saturated sum of two input values.');text(10,60,'NXP 2022');text(10,45,'1.0');text(10,30,'20-Apr-2022');
  f16Out : Outport
  wires:
  MLIB_MacSat_SF/1 -> f16Out/1
  f16In3/1 -> MLIB_MacSat_SF/3
  f16In2/1 -> MLIB_MacSat_SF/2
  f16In1/1 -> MLIB_MacSat_SF/1

== system ammclib_bam_S32K3xx/MLIB/F16/MLIB_Mac_F16 ==
  f16In1 : Inport  OutDataTypeStr=int16
  f16In2 : Inport  Port=2  OutDataTypeStr=int16
  f16In3 : Inport  Port=3  OutDataTypeStr=int16
  MLIB_Mac_SF : S-Function  FunctionName=MLIB_Mac_SF_F16  SFunctionDeploymentMode=off  EnableBusSupport=off
  copyright : Subsystem
      mask Display: text(10,90,'FILE:');text(10,75,'DESRIPTION:');text(10,60,'COPYRIGHT:');text(10,45,'VERSION:');text(10,30,'DATE:')
  copyright2 : Subsystem
      mask Display: text(10,90,'MLIB_Mac_BAM_F16.slx');text(10,75,'Multiply-accumulte.');text(10,60,'NXP 2022');text(10,45,'1.0');text(10,30,'20-Apr-2022');
  f16Out : Outport
  wires:
  MLIB_Mac_SF/1 -> f16Out/1
  f16In3/1 -> MLIB_Mac_SF/3
  f16In2/1 -> MLIB_Mac_SF/2
  f16In1/1 -> MLIB_Mac_SF/1

== system ammclib_bam_S32K3xx/MLIB/F16/MLIB_Mnac_F16 ==
  f16In1 : Inport  OutDataTypeStr=int16
  f16In2 : Inport  Port=2  OutDataTypeStr=int16
  f16In3 : Inport  Port=3  OutDataTypeStr=int16
  MLIB_Mnac_SF : S-Function  FunctionName=MLIB_Mnac_SF_F16  SFunctionDeploymentMode=off  EnableBusSupport=off
  copyright : Subsystem
      mask Display: text(10,90,'FILE:');text(10,75,'DESRIPTION:');text(10,60,'COPYRIGHT:');text(10,45,'VERSION:');text(10,30,'DATE:')
  copyright2 : Subsystem
      mask Display: text(10,90,'MLIB_Mnac_BAM_F16.slx');text(10,75,'Unsaturated multiply-negative-accumulate.');text(10,60,'NXP 2022');text(10,45,'1.0');text(10,30,'20-Apr-2022');
  f16Out : Outport
  wires:
  MLIB_Mnac_SF/1 -> f16Out/1
  f16In3/1 -> MLIB_Mnac_SF/3
  f16In2/1 -> MLIB_Mnac_SF/2
  f16In1/1 -> MLIB_Mnac_SF/1

== system ammclib_bam_S32K3xx/MLIB/F16/MLIB_Msu_F16 ==
  f16In1 : Inport  OutDataTypeStr=int16
  f16In2 : Inport  Port=2  OutDataTypeStr=int16
  f16In3 : Inport  Port=3  OutDataTypeStr=int16
  MLIB_Msu_SF : S-Function  FunctionName=MLIB_Msu_SF_F16  SFunctionDeploymentMode=off  EnableBusSupport=off
  copyright : Subsystem
      mask Display: text(10,90,'FILE:');text(10,75,'DESRIPTION:');text(10,60,'COPYRIGHT:');text(10,45,'VERSION:');text(10,30,'DATE:')
  copyright2 : Subsystem
      mask Display: text(10,90,'MLIB_Msu_BAM_F16.slx');text(10,75,'Unsaturated multiply-subtract-from.');text(10,60,'NXP 2022');text(10,45,'1.0');text(10,30,'20-Apr-2022');
  f16Out : Outport
  wires:
  MLIB_Msu_SF/1 -> f16Out/1
  f16In3/1 -> MLIB_Msu_SF/3
  f16In2/1 -> MLIB_Msu_SF/2
  f16In1/1 -> MLIB_Msu_SF/1

== system ammclib_bam_S32K3xx/MLIB/F16/MLIB_MulSat_F16 ==
  f16In1 : Inport  OutDataTypeStr=int16
  f16In2 : Inport  Port=2  OutDataTypeStr=int16
  MLIB_MulSat_SF : S-Function  FunctionName=MLIB_MulSat_SF_F16  SFunctionDeploymentMode=off  EnableBusSupport=off
  copyright : Subsystem
      mask Display: text(10,90,'FILE:');text(10,75,'DESRIPTION:');text(10,60,'COPYRIGHT:');text(10,45,'VERSION:');text(10,30,'DATE:')
  copyright2 : Subsystem
      mask Display: text(10,90,'MLIB_MulSat_BAM_F16.slx');text(10,75,'Saturated multiplication.');text(10,60,'NXP 2022');text(10,45,'1.0');text(10,30,'20-Apr-2022');
  f16Out : Outport
  wires:
  MLIB_MulSat_SF/1 -> f16Out/1
  f16In2/1 -> MLIB_MulSat_SF/2
  f16In1/1 -> MLIB_MulSat_SF/1

== system ammclib_bam_S32K3xx/MLIB/F16/MLIB_Mul_F16 ==
  f16In1 : Inport  OutDataTypeStr=int16
  f16In2 : Inport  Port=2  OutDataTypeStr=int16
  MLIB_Mul_SF : S-Function  FunctionName=MLIB_Mul_SF_F16  SFunctionDeploymentMode=off  EnableBusSupport=off
  copyright : Subsystem
      mask Display: text(10,90,'FILE:');text(10,75,'DESRIPTION:');text(10,60,'COPYRIGHT:');text(10,45,'VERSION:');text(10,30,'DATE:')
  copyright2 : Subsystem
      mask Display: text(10,90,'MLIB_Mul_BAM_F16.slx');text(10,75,'Unsaturated multiplication.');text(10,60,'NXP 2022');text(10,45,'1.0');text(10,30,'20-Apr-2022');
  f16Out : Outport
  wires:
  MLIB_Mul_SF/1 -> f16Out/1
  f16In2/1 -> MLIB_Mul_SF/2
  f16In1/1 -> MLIB_Mul_SF/1

== system ammclib_bam_S32K3xx/MLIB/F16/MLIB_NegSat_F16 ==
  f16In : Inport  OutDataTypeStr=int16
  MLIB_NegSat_SF : S-Function  FunctionName=MLIB_NegSat_SF_F16  SFunctionDeploymentMode=off  EnableBusSupport=off
  copyright : Subsystem
      mask Display: text(10,90,'FILE:');text(10,75,'DESRIPTION:');text(10,60,'COPYRIGHT:');text(10,45,'VERSION:');text(10,30,'DATE:')
  copyright2 : Subsystem
      mask Display: text(10,90,'MLIB_NegSat_BAM_F16.slx');text(10,75,'Saturated negation.');text(10,60,'NXP 2022');text(10,45,'1.0');text(10,30,'20-Apr-2022');
  f16Out : Outport
  wires:
  MLIB_NegSat_SF/1 -> f16Out/1
  f16In/1 -> MLIB_NegSat_SF/1

== system ammclib_bam_S32K3xx/MLIB/F16/MLIB_Neg_F16 ==
  f16In : Inport  OutDataTypeStr=int16
  MLIB_Neg_SF : S-Function  FunctionName=MLIB_Neg_SF_F16  SFunctionDeploymentMode=off  EnableBusSupport=off
  copyright : Subsystem
      mask Display: text(10,90,'FILE:');text(10,75,'DESRIPTION:');text(10,60,'COPYRIGHT:');text(10,45,'VERSION:');text(10,30,'DATE:')
  copyright2 : Subsystem
      mask Display: text(10,90,'MLIB_Neg_BAM_F16.slx');text(10,75,'Unsaturated negation.');text(10,60,'NXP 2022');text(10,45,'1.0');text(10,30,'20-Apr-2022');
  f16Out : Outport
  wires:
  MLIB_Neg_SF/1 -> f16Out/1
  f16In/1 -> MLIB_Neg_SF/1

== system ammclib_bam_S32K3xx/MLIB/F16/MLIB_Norm_F16 ==
  f16In : Inport  OutDataTypeStr=int16
  MLIB_Norm_SF : S-Function  FunctionName=MLIB_Norm_SF_F16  SFunctionDeploymentMode=off  EnableBusSupport=off
  copyright : Subsystem
      mask Display: text(10,90,'FILE:');text(10,75,'DESRIPTION:');text(10,60,'COPYRIGHT:');text(10,45,'VERSION:');text(10,30,'DATE:')
  copyright2 : Subsystem
      mask Display: text(10,90,'MLIB_Norm_BAM_F16.slx');text(10,75,'Normalization of the input value.');text(10,60,'NXP 2022');text(10,45,'1.0');text(10,30,'20-Apr-2022');
  u16Out : Outport
  wires:
  MLIB_Norm_SF/1 -> u16Out/1
  f16In/1 -> MLIB_Norm_SF/1

== system ammclib_bam_S32K3xx/MLIB/F16/MLIB_RndSat_F16F32 ==
  f32In : Inport  OutDataTypeStr=int32
  MLIB_RndSat_SF : S-Function  FunctionName=MLIB_RndSat_SF_F16F32  SFunctionDeploymentMode=off  EnableBusSupport=off
  copyright : Subsystem
      mask Display: text(10,90,'FILE:');text(10,75,'DESRIPTION:');text(10,60,'COPYRIGHT:');text(10,45,'VERSION:');text(10,30,'DATE:')
  copyright2 : Subsystem
      mask Display: text(10,90,'MLIB_RndSat_BAM_F16F32.slx');text(10,75,'Saturated round to nearest.');text(10,60,'NXP 2022');text(10,45,'1.0');text(10,30,'20-Apr-2022');
  f16Out : Outport
  wires:
  MLIB_RndSat_SF/1 -> f16Out/1
  f32In/1 -> MLIB_RndSat_SF/1

== system ammclib_bam_S32K3xx/MLIB/F16/MLIB_Round_F16 ==
  f16In1 : Inport  OutDataTypeStr=int16
  u16In2 : Inport  Port=2  OutDataTypeStr=uint16
  MLIB_Round_SF : S-Function  FunctionName=MLIB_Round_SF_F16  SFunctionDeploymentMode=off  EnableBusSupport=off
  copyright : Subsystem
      mask Display: text(10,90,'FILE:');text(10,75,'DESRIPTION:');text(10,60,'COPYRIGHT:');text(10,45,'VERSION:');text(10,30,'DATE:')
  copyright2 : Subsystem
      mask Display: text(10,90,'MLIB_Round_BAM_F16.slx');text(10,75,'Round the first input value.');text(10,60,'NXP 2022');text(10,45,'1.0');text(10,30,'20-Apr-2022');
  f16Out : Outport
  wires:
  MLIB_Round_SF/1 -> f16Out/1
  u16In2/1 -> MLIB_Round_SF/2
  f16In1/1 -> MLIB_Round_SF/1

== system ammclib_bam_S32K3xx/MLIB/F16/MLIB_ShBiSat_F16 ==
  f16In1 : Inport  OutDataTypeStr=int16
  s16In2 : Inport  Port=2  OutDataTypeStr=int16
  MLIB_ShBiSat_SF : S-Function  FunctionName=MLIB_ShBiSat_SF_F16  SFunctionDeploymentMode=off  EnableBusSupport=off
  copyright : Subsystem
      mask Display: text(10,90,'FILE:');text(10,75,'DESRIPTION:');text(10,60,'COPYRIGHT:');text(10,45,'VERSION:');text(10,30,'DATE:')
  copyright2 : Subsystem
      mask Display: text(10,90,'MLIB_ShBiSat_BAM_F16.slx');text(10,75,'Saturated bidirectional shift.');text(10,60,'NXP 2022');text(10,45,'1.0');text(10,30,'20-Apr-2022');
  f16Out : Outport
  wires:
  MLIB_ShBiSat_SF/1 -> f16Out/1
  s16In2/1 -> MLIB_ShBiSat_SF/2
  f16In1/1 -> MLIB_ShBiSat_SF/1

== system ammclib_bam_S32K3xx/MLIB/F16/MLIB_ShBi_F16 ==
  f16In1 : Inport  OutDataTypeStr=int16
  s16In2 : Inport  Port=2  OutDataTypeStr=int16
  MLIB_ShBi_SF : S-Function  FunctionName=MLIB_ShBi_SF_F16  SFunctionDeploymentMode=off  EnableBusSupport=off
  copyright : Subsystem
      mask Display: text(10,90,'FILE:');text(10,75,'DESRIPTION:');text(10,60,'COPYRIGHT:');text(10,45,'VERSION:');text(10,30,'DATE:')
  copyright2 : Subsystem
      mask Display: text(10,90,'MLIB_ShBi_BAM_F16.slx');text(10,75,'Unsaturated bidirectional shift.');text(10,60,'NXP 2022');text(10,45,'1.0');text(10,30,'20-Apr-2022');
  f16Out : Outport
  wires:
  MLIB_ShBi_SF/1 -> f16Out/1
  s16In2/1 -> MLIB_ShBi_SF/2
  f16In1/1 -> MLIB_ShBi_SF/1

== system ammclib_bam_S32K3xx/MLIB/F16/MLIB_ShLSat_F16 ==
  f16In1 : Inport  OutDataTypeStr=int16
  u16In2 : Inport  Port=2  OutDataTypeStr=uint16
  MLIB_ShLSat_SF : S-Function  FunctionName=MLIB_ShLSat_SF_F16  SFunctionDeploymentMode=off  EnableBusSupport=off
  copyright : Subsystem
      mask Display: text(10,90,'FILE:');text(10,75,'DESRIPTION:');text(10,60,'COPYRIGHT:');text(10,45,'VERSION:');text(10,30,'DATE:')
  copyright2 : Subsystem
      mask Display: text(10,90,'MLIB_ShLSat_BAM_F16.slx');text(10,75,'Saturated shift left.');text(10,60,'NXP 2022');text(10,45,'1.0');text(10,30,'20-Apr-2022');
  f16Out : Outport
  wires:
  MLIB_ShLSat_SF/1 -> f16Out/1
  u16In2/1 -> MLIB_ShLSat_SF/2
  f16In1/1 -> MLIB_ShLSat_SF/1

== system ammclib_bam_S32K3xx/MLIB/F16/MLIB_ShL_F16 ==
  f16In1 : Inport  OutDataTypeStr=int16
  u16In2 : Inport  Port=2  OutDataTypeStr=uint16
  MLIB_ShL_SF : S-Function  FunctionName=MLIB_ShL_SF_F16  SFunctionDeploymentMode=off  EnableBusSupport=off
  copyright : Subsystem
      mask Display: text(10,90,'FILE:');text(10,75,'DESRIPTION:');text(10,60,'COPYRIGHT:');text(10,45,'VERSION:');text(10,30,'DATE:')
  copyright2 : Subsystem
      mask Display: text(10,90,'MLIB_ShL_BAM_F16.slx');text(10,75,'Unsaturated shift left.');text(10,60,'NXP 2022');text(10,45,'1.0');text(10,30,'20-Apr-2022');
  f16Out : Outport
  wires:
  MLIB_ShL_SF/1 -> f16Out/1
  u16In2/1 -> MLIB_ShL_SF/2
  f16In1/1 -> MLIB_ShL_SF/1

== system ammclib_bam_S32K3xx/MLIB/F16/MLIB_ShR_F16 ==
  f16In1 : Inport  OutDataTypeStr=int16
  u16In2 : Inport  Port=2  OutDataTypeStr=uint16
  MLIB_ShR_SF : S-Function  FunctionName=MLIB_ShR_SF_F16  SFunctionDeploymentMode=off  EnableBusSupport=off
  copyright : Subsystem
      mask Display: text(10,90,'FILE:');text(10,75,'DESRIPTION:');text(10,60,'COPYRIGHT:');text(10,45,'VERSION:');text(10,30,'DATE:')
  copyright2 : Subsystem
      mask Display: text(10,90,'MLIB_ShR_BAM_F16.slx');text(10,75,'Unsaturated shift right.');text(10,60,'NXP 2022');text(10,45,'1.0');text(10,30,'20-Apr-2022');
  f16Out : Outport
  wires:
  MLIB_ShR_SF/1 -> f16Out/1
  u16In2/1 -> MLIB_ShR_SF/2
  f16In1/1 -> MLIB_ShR_SF/1

== system ammclib_bam_S32K3xx/MLIB/F16/MLIB_SubSat_F16 ==
  f16In1 : Inport  OutDataTypeStr=int16
  f16In2 : Inport  Port=2  OutDataTypeStr=int16
  MLIB_SubSat_SF : S-Function  FunctionName=MLIB_SubSat_SF_F16  SFunctionDeploymentMode=off  EnableBusSupport=off
  copyright : Subsystem
      mask Display: text(10,90,'FILE:');text(10,75,'DESRIPTION:');text(10,60,'COPYRIGHT:');text(10,45,'VERSION:');text(10,30,'DATE:')
  copyright2 : Subsystem
      mask Display: text(10,90,'MLIB_SubSat_BAM_F16.slx');text(10,75,'Saturated subtraction.');text(10,60,'NXP 2022');text(10,45,'1.0');text(10,30,'20-Apr-2022');
  f16Out : Outport
  wires:
  MLIB_SubSat_SF/1 -> f16Out/1
  f16In2/1 -> MLIB_SubSat_SF/2
  f16In1/1 -> MLIB_SubSat_SF/1

== system ammclib_bam_S32K3xx/MLIB/F16/MLIB_Sub_F16 ==
  f16In1 : Inport  OutDataTypeStr=int16
  f16In2 : Inport  Port=2  OutDataTypeStr=int16
  MLIB_Sub_SF : S-Function  FunctionName=MLIB_Sub_SF_F16  SFunctionDeploymentMode=off  EnableBusSupport=off
  copyright : Subsystem
      mask Display: text(10,90,'FILE:');text(10,75,'DESRIPTION:');text(10,60,'COPYRIGHT:');text(10,45,'VERSION:');text(10,30,'DATE:')
  copyright2 : Subsystem
      mask Display: text(10,90,'MLIB_Sub_BAM_F16.slx');text(10,75,'Unsaturated subtraction.');text(10,60,'NXP 2022');text(10,45,'1.0');text(10,30,'20-Apr-2022');
  f16Out : Outport
  wires:
  MLIB_Sub_SF/1 -> f16Out/1
  f16In2/1 -> MLIB_Sub_SF/2
  f16In1/1 -> MLIB_Sub_SF/1

== system ammclib_bam_S32K3xx/MLIB/F16/MLIB_VAdd_F16 ==
  f16In1 : Inport  OutDataTypeStr=Bus: SWLIBS_2Syst_F16  BusOutputAsStruct=on
  f16In2 : Inport  Port=2  OutDataTypeStr=Bus: SWLIBS_2Syst_F16  BusOutputAsStruct=on
  MLIB_VAdd_SF : S-Function  FunctionName=MLIB_VAdd_SF_F16  SFunctionDeploymentMode=off  EnableBusSupport=off
  copyright : Subsystem
      mask Display: text(10,90,'FILE:');text(10,75,'DESRIPTION:');text(10,60,'COPYRIGHT:');text(10,45,'VERSION:');text(10,30,'DATE:')
  copyright2 : Subsystem
      mask Display: text(10,90,'MLIB_VAdd_BAM_F16.slx');text(10,75,'Vector addition.');text(10,60,'NXP 2022');text(10,45,'1.0');text(10,30,'20-Apr-2022');
  f16Out : Outport
  wires:
  MLIB_VAdd_SF/1 -> f16Out/1
  f16In2/1 -> MLIB_VAdd_SF/2
  f16In1/1 -> MLIB_VAdd_SF/1

== system ammclib_bam_S32K3xx/MLIB/F16/MLIB_VMac_F16 ==
  f16In1 : Inport  OutDataTypeStr=int16
  f16In2 : Inport  Port=2  OutDataTypeStr=int16
  f16In3 : Inport  Port=3  OutDataTypeStr=int16
  f16In4 : Inport  Port=4  OutDataTypeStr=int16
  MLIB_VMac_SF : S-Function  FunctionName=MLIB_VMac_SF_F16  SFunctionDeploymentMode=off  EnableBusSupport=off
  copyright : Subsystem
      mask Display: text(10,90,'FILE:');text(10,75,'DESRIPTION:');text(10,60,'COPYRIGHT:');text(10,45,'VERSION:');text(10,30,'DATE:')
  copyright2 : Subsystem
      mask Display: text(10,90,'MLIB_VMac_BAM_F16.slx');text(10,75,'Dot product of 2-element vectors with saturated multiplication and modulo accumulation.');text(10,60,'NXP 2022');text(10,45,'1.0');text(10,30,'20-Apr-2022');
  f16Out : Outport
  wires:
  MLIB_VMac_SF/1 -> f16Out/1
  f16In4/1 -> MLIB_VMac_SF/4
  f16In3/1 -> MLIB_VMac_SF/3
  f16In2/1 -> MLIB_VMac_SF/2
  f16In1/1 -> MLIB_VMac_SF/1

== system ammclib_bam_S32K3xx/MLIB/F16/MLIB_VScale_F16 ==
  f16InVec : Inport  OutDataTypeStr=Bus: SWLIBS_2Syst_F16  BusOutputAsStruct=on
  f16InScale : Inport  Port=2  OutDataTypeStr=int16
  MLIB_VScale_SF : S-Function  FunctionName=MLIB_VScale_SF_F16  SFunctionDeploymentMode=off  EnableBusSupport=off
  copyright : Subsystem
      mask Display: text(10,90,'FILE:');text(10,75,'DESRIPTION:');text(10,60,'COPYRIGHT:');text(10,45,'VERSION:');text(10,30,'DATE:')
  copyright2 : Subsystem
      mask Display: text(10,90,'MLIB_VScale_BAM_F16.slx');text(10,75,'Multiplication of a vector and scalar.');text(10,60,'NXP 2022');text(10,45,'1.0');text(10,30,'20-Apr-2022');
  f16OutVec : Outport
  wires:
  MLIB_VScale_SF/1 -> f16OutVec/1
  f16InScale/1 -> MLIB_VScale_SF/2
  f16InVec/1 -> MLIB_VScale_SF/1

== system ammclib_bam_S32K3xx/MLIB/F16/MLIB_VSub_F16 ==
  f16In1 : Inport  OutDataTypeStr=Bus: SWLIBS_2Syst_F16  BusOutputAsStruct=on
  f16In2 : Inport  Port=2  OutDataTypeStr=Bus: SWLIBS_2Syst_F16  BusOutputAsStruct=on
  MLIB_VSub_SF : S-Function  FunctionName=MLIB_VSub_SF_F16  SFunctionDeploymentMode=off  EnableBusSupport=off
  copyright : Subsystem
      mask Display: text(10,90,'FILE:');text(10,75,'DESRIPTION:');text(10,60,'COPYRIGHT:');text(10,45,'VERSION:');text(10,30,'DATE:')
  copyright2 : Subsystem
      mask Display: text(10,90,'MLIB_VSub_BAM_F16.slx');text(10,75,'Vector substraction.');text(10,60,'NXP 2022');text(10,45,'1.0');text(10,30,'20-Apr-2022');
  f16Out : Outport
  wires:
  MLIB_VSub_SF/1 -> f16Out/1
  f16In2/1 -> MLIB_VSub_SF/2
  f16In1/1 -> MLIB_VSub_SF/1

== system ammclib_bam_S32K3xx/MLIB/F32/MLIB_AbsSat_F32 ==
  f32In : Inport  OutDataTypeStr=int32
  MLIB_AbsSat_SF : S-Function  FunctionName=MLIB_AbsSat_SF_F32  SFunctionDeploymentMode=off  EnableBusSupport=off
  copyright : Subsystem
      mask Display: text(10,90,'FILE:');text(10,75,'DESRIPTION:');text(10,60,'COPYRIGHT:');text(10,45,'VERSION:');text(10,30,'DATE:')
  copyright2 : Subsystem
      mask Display: text(10,90,'MLIB_AbsSat_BAM_F32.slx');text(10,75,'Saturated absolute value.');text(10,60,'NXP 2022');text(10,45,'1.0');text(10,30,'20-Apr-2022');
  f32Out : Outport
  wires:
  MLIB_AbsSat_SF/1 -> f32Out/1
  f32In/1 -> MLIB_AbsSat_SF/1

== system ammclib_bam_S32K3xx/MLIB/F32/MLIB_Abs_F32 ==
  f32In : Inport  OutDataTypeStr=int32
  MLIB_Abs_SF : S-Function  FunctionName=MLIB_Abs_SF_F32  SFunctionDeploymentMode=off  EnableBusSupport=off
  copyright : Subsystem
      mask Display: text(10,90,'FILE:');text(10,75,'DESRIPTION:');text(10,60,'COPYRIGHT:');text(10,45,'VERSION:');text(10,30,'DATE:')
  copyright2 : Subsystem
      mask Display: text(10,90,'MLIB_Abs_BAM_F32.slx');text(10,75,'Unsaturated absolute value.');text(10,60,'NXP 2022');text(10,45,'1.0');text(10,30,'20-Apr-2022');
  f32Out : Outport
  wires:
  MLIB_Abs_SF/1 -> f32Out/1
  f32In/1 -> MLIB_Abs_SF/1

== system ammclib_bam_S32K3xx/MLIB/F32/MLIB_AddSat_F32 ==
  f32In1 : Inport  OutDataTypeStr=int32
  f32In2 : Inport  Port=2  OutDataTypeStr=int32
  MLIB_AddSat_SF : S-Function  FunctionName=MLIB_AddSat_SF_F32  SFunctionDeploymentMode=off  EnableBusSupport=off
  copyright : Subsystem
      mask Display: text(10,90,'FILE:');text(10,75,'DESRIPTION:');text(10,60,'COPYRIGHT:');text(10,45,'VERSION:');text(10,30,'DATE:')
  copyright2 : Subsystem
      mask Display: text(10,90,'MLIB_AddSat_BAM_F32.slx');text(10,75,'Saturated addition.');text(10,60,'NXP 2022');text(10,45,'1.0');text(10,30,'20-Apr-2022');
  f32Out : Outport
  wires:
  MLIB_AddSat_SF/1 -> f32Out/1
  f32In2/1 -> MLIB_AddSat_SF/2
  f32In1/1 -> MLIB_AddSat_SF/1

== system ammclib_bam_S32K3xx/MLIB/F32/MLIB_Add_F32 ==
  f32In1 : Inport  OutDataTypeStr=int32
  f32In2 : Inport  Port=2  OutDataTypeStr=int32
  MLIB_Add_SF : S-Function  FunctionName=MLIB_Add_SF_F32  SFunctionDeploymentMode=off  EnableBusSupport=off
  copyright : Subsystem
      mask Display: text(10,90,'FILE:');text(10,75,'DESRIPTION:');text(10,60,'COPYRIGHT:');text(10,45,'VERSION:');text(10,30,'DATE:')
  copyright2 : Subsystem
      mask Display: text(10,90,'MLIB_Add_BAM_F32.slx');text(10,75,'Unsaturated addition.');text(10,60,'NXP 2022');text(10,45,'1.0');text(10,30,'20-Apr-2022');
  f32Out : Outport
  wires:
  MLIB_Add_SF/1 -> f32Out/1
  f32In2/1 -> MLIB_Add_SF/2
  f32In1/1 -> MLIB_Add_SF/1

== system ammclib_bam_S32K3xx/MLIB/F32/MLIB_ConvertPU_F32F16 ==
  f16In : Inport  OutDataTypeStr=int16
  MLIB_ConvertPU_SF : S-Function  FunctionName=MLIB_ConvertPU_SF_F32F16  SFunctionDeploymentMode=off  EnableBusSupport=off
  copyright : Subsystem
      mask Display: text(10,90,'FILE:');text(10,75,'DESRIPTION:');text(10,60,'COPYRIGHT:');text(10,45,'VERSION:');text(10,30,'DATE:')
  copyright2 : Subsystem
      mask Display: text(10,90,'MLIB_ConvertPU_BAM_F32F16.slx');text(10,75,'Converts the input value to a different representation.');text(10,60,'NXP 2022');text(10,45,'1.0');text(10,30,'20-Apr-2022');
  f32Out : Outport
  wires:
  MLIB_ConvertPU_SF/1 -> f32Out/1
  f16In/1 -> MLIB_ConvertPU_SF/1
